simulink model "LogicalOperator_TestGen8"  (R2017b)
settings: Solver=FixedStepDiscrete  StartTime=0.0  StopTime=10.0  RelTol=1e-3
undefined symbols (not defined in the file): Block_TestLib, trigger
settings Model: Creator=ktrinh  LastModifiedBy=ktrinh
settings DebuggingCC: ParameterOverflowMsg=none

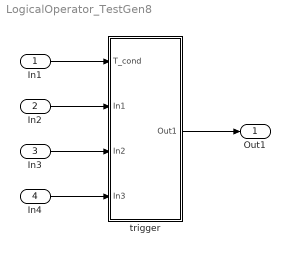
== system LogicalOperator_TestGen8 ==
  In1 : Inport
  In2 : Inport  Port=2
  In3 : Inport  Port=3
  In4 : Inport  Port=4
  trigger : Subsystem  AncestorBlock=Block_TestLib/trigger
  Out1 : Outport
  wires:
  In1/1 -> trigger/1(T_cond)
  In2/1 -> trigger/2(In1)
  In3/1 -> trigger/3(In2)
  In4/1 -> trigger/4(In3)
  trigger/1(Out1) -> Out1/1

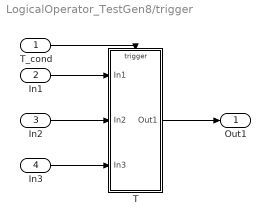
== system LogicalOperator_TestGen8/trigger ==
  T_cond : Inport  OutDataTypeStr=boolean
  In1 : Inport  Port=2
  In2 : Inport  Port=3
  In3 : Inport  Port=4
  T : Subsystem  TreatAsAtomicUnit=on
  Out1 : Outport
  wires:
  T_cond/1 -> T/Trigger
  In1/1 -> T/1(In1)
  In2/1 -> T/2(In2)
  In3/1 -> T/3(In3)
  T/1(Out1) -> Out1/1

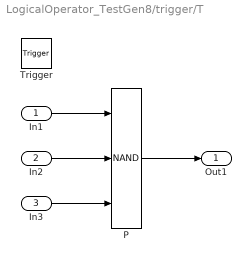
== system LogicalOperator_TestGen8/trigger/T ==
  In1 : Inport  OutDataTypeStr=boolean  PortDimensions=1
  In2 : Inport  Port=2  OutDataTypeStr=boolean  PortDimensions=1
  In3 : Inport  Port=3  OutDataTypeStr=boolean  PortDimensions=1
  Trigger : TriggerPort  VariantControl=Variant
  P : Logic  Operator=NAND  Inputs=3  OutDataTypeStr=boolean
  Out1 : Outport
  wires:
  In1/1 -> P/1
  In2/1 -> P/2
  In3/1 -> P/3
  P/1 -> Out1/1
